simulink model "first_part"  (R2020b)
settings: Solver=ode45  StartTime=0.0  StopTime=10.0  RelTol=1e-3
model workspace (MAT data in the model file):
  auto = 0.00448959494016
  u = 1
settings Model: Creator=ilya-  LastModifiedBy=Le tueur

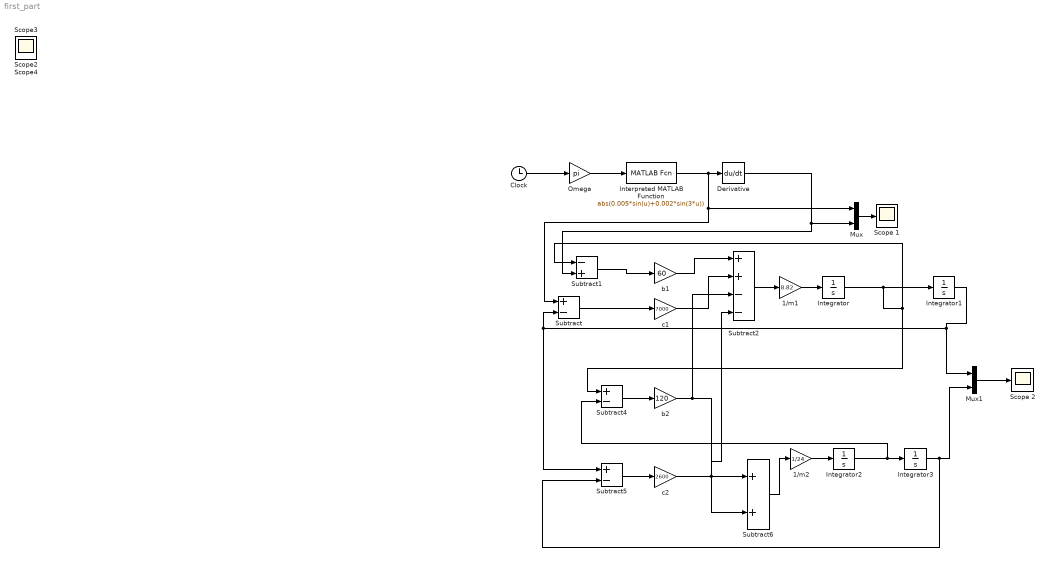
== system first_part ==
  1/m1 : Gain  Gain=8.82
  1/m2 : Gain  Gain=1/24
  Clock : Clock
  Derivative : Derivative
  Integrator{,1..3} (4 alike) : Integrator
  Interpreted MATLAB Function : MATLABFcn  MATLABFcn=abs(0.005*sin(u)+0.002*sin(3*u))  OutputSignalType=real
  Mux : Mux  Inputs=2
  Mux1 : Mux  Inputs=2
  Omega : Gain  Gain=pi
  Scope 1 : Scope
  Scope 2 : Scope
  Subtract : Sum  Inputs=+-
  Subtract1 : Sum  Inputs=-+
  Subtract2 : Sum  Inputs=++--
  Subtract4 : Sum  Inputs=+-
  Subtract5 : Sum  Inputs=+-
  Subtract6 : Sum
  b1 : Gain  Gain=60
  b2 : Gain  Gain=120
  c1 : Gain  Gain=7000
  c2 : Gain  Gain=2600
  Scope2 : Scope
  Scope3 : Scope
  Scope4 : Scope
  wires:
  Clock/1 -> Omega/1
  Omega/1 -> Interpreted MATLAB Function/1
  Interpreted MATLAB Function/1 -> Mux/1, Subtract/1, Derivative/1
  Mux/1 -> Scope 1/1
  Subtract/1 -> c1/1
  Subtract1/1 -> b1/1
  b1/1 -> Subtract2/1
  c1/1 -> Subtract2/2
  Subtract2/1 -> 1/m1/1
  1/m1/1 -> Integrator/1
  Integrator/1 -> Integrator1/1, Subtract4/1, Subtract1/1
  Derivative/1 -> Mux/2, Subtract1/2
  Subtract4/1 -> b2/1
  Subtract5/1 -> c2/1
  c2/1 -> Subtract2/4, Subtract6/2
  Mux1/1 -> Scope 2/1
  1/m2/1 -> Integrator2/1
  Subtract6/1 -> 1/m2/1
  Integrator2/1 -> Subtract4/2, Integrator3/1
  b2/1 -> Subtract2/3, Subtract6/1
  Integrator3/1 -> Subtract5/2, Mux1/2
  Integrator1/1 -> Mux1/1, Subtract5/1, Subtract/2
